simulink model "CiEngineController"  (R2017b)
settings: Solver=ode4  StartTime=0.0  StopTime=inf  FixedStep=.01  RelTol=1e-3  EnableMultiTasking=on
model workspace (MAT data in the model file):
  AFRStoich = 14.6
  CatLightOffTime = 0
  Cps = 2
  DesiredIdleSpeed = 750
  EGRAP_FFD = [31.29325855 19.51543729 10.79128083 10.46559436 21.98337597 33.12149522 39.82825957 47.90500302 59.68238122 67.88485049 66.83182002 60.43695561 ... (225 elements, 15x15)]
  EngStopStartEnable = 1
  EngStopTime = Simulink.Parameter
  EngStopTime.Value = 5
  EngStopTime.DataType = 'auto'
  EngStopTime.Dimensions = [1 1]
  InjSlp = 6.45161290323
  NCyl = 4
  Pstd = 101325
  Rair = 287.05
  Speed_bp = [1000 1285.71428571 1571.42857143 1857.14285714 2142.85714286 2428.57142857 2714.28571429 3000 3285.71428571 3571.42857143 3857.14285714 4142.85714286 4428.57142857 4714.28571429 5000]
  TQ_Simple = [0 10.3191931725 31.7529891947 50.7995054407 67.7372596761 83.6143476896 99.4031459341 115.400676238 131.426595678 147.347834106 163.740159238 181.145988166 ... (225 elements, 15x15)]
  TQ_Simple_FuelMass_bp = [0 3.5714 7.1429 10.7143 14.2857 17.8571 21.4286 25 28.5714 32.1429 35.7143 39.2857 42.8571 46.4286 50]
  TQ_Simple_Speed_bp = [1000 1410.7143 1821.4286 2232.1429 2642.8571 3053.5714 3464.2857 3875 4285.7143 4696.4286 5107.1429 5517.8571 5928.5714 6339.2857 6750]
  Torque_bp = [10 26.4285714286 42.8571428571 59.2857142857 75.7142857143 92.1428571429 108.571428571 125 141.428571429 157.857142857 174.285714286 190.714285714 207.142857143 223.571428571 240]
  Ts = Simulink.Parameter
  Ts.Value = 0.01
  Ts.DataType = 'auto'
  Ts.Dimensions = [1 1]
  Tstd = 293.15
  VGTPOS_FFD = [0.726426588 0.790379264 0.744536274 0.574005744 0.384541159 0.290234957 0.352244481 0.466398697 0.509945722 0.516364986 0.532540266 0.566278183 ... (225 elements, 15x15)]
  Vd = 0.0015
  VolEffEngSpdBpt = [1000 1285.71428571 1571.42857143 1857.14285714 2142.85714286 2428.57142857 2714.28571429 3000 3285.71428571 3571.42857143 3857.14285714 4142.85714286 4428.57142857 4714.28571429 5000]
  VolEffMapBpt = [95 100.344827586 105.689655172 111.034482759 116.379310345 121.724137931 127.068965517 132.413793103 137.75862069 143.103448276 148.448275862 153.793103448 159.137931034 164.482758621 169.827586207 175.172413793 180.517241379 185.862068966 191.206896552 196.551724138 201.896551724 207.24137931 212.586206897 217.931034483 223.275862069 228.620689655 233.965517241 239.310344828 244.655172414 250]
  VolEffTbl = [0.954646224834 0.927678310575 0.901063682417 0.875710037198 0.852450535311 0.831986822876 0.814844392337 0.80134438932 0.791593989181 0.785495277781 0.782770492696 0.782999798686 ... (450 elements, 30x15)]
  f_egr_stdflow = [0 0 0 0 0 0 0 0 0 0 0 0 ... (225 elements, 15x15)]
  f_egr_stdflow_egrap_bpt = [0 7.14285714286 14.2857142857 21.4285714286 28.5714285714 35.7142857143 42.8571428571 50 57.1428571429 64.2857142857 71.4285714286 78.5714285714 85.7142857143 92.8571428571 100]
  f_egr_stdflow_pr_bpt = [0.5 0.535714285714 0.571428571429 0.607142857143 0.642857142857 0.678571428571 0.714285714286 0.75 0.785714285714 0.821428571429 0.857142857143 0.892857142857 0.928571428571 0.964285714286 1]
  f_f_tot_n_bpt = [1000 1285.71428571 1571.42857143 1857.14285714 2142.85714286 2428.57142857 2714.28571429 3000 3285.71428571 3571.42857143 3857.14285714 4142.85714286 4428.57142857 4714.28571429 5000]
  f_f_tot_tq_bpt = [0 10 26.42857143 42.85714286 59.28571429 75.71428571 92.14285714 108.5714286 125 141.4285714 157.8571429 174.2857143 190.7142857 207.1428571 223.5714286 240]
  f_fcmd_tot = [7.10205580862 7.10205580862 10.8378455551 14.7842820505 18.9326887052 24.470710663 31.0466929023 35.2080453505 35.2080451224 35.2080448944 35.2080461396 35.2080459117 ... (240 elements, 16x15)]
  f_fric_temp_bpt = [275 277 279 281 283 285 287 289 291 293 295 297 299 301 303 305 307 309 311 313 315 317 319 321 323 325 327 329 331 333 335 337 339 341 343 345 347 349 351 353 355 357 359 361 363 365]
  f_fric_temp_mod = [3.986 2.616 2.132 1.946 1.839 1.747 1.672 1.608 1.551 1.499 1.462 1.415 1.363 1.314 1.275 1.248 1.223 1.195 1.173 1.15 1.134 1.113 1.097 1.082 1.065 1.051 1.039 1.025 1.01 1.001 0.9907 0.9802 0.9699 0.9595 0.9593 0.954 0.9415 0.9368 0.9285 0.923 0.9185 0.9093 0.9018 0.8989 0.8965 0.887]
  f_main_soi = [1.11993303174 2.12125793974 1.25580736048 -0.781894253933 -4.17418882707 -6.2159077095 -4.45741400372 -3.71779708796 -4.35326957016 -4.73674822365 -4.93672626877 -4.76868482083 ... (225 elements, 15x15)]
  f_main_soi_f_bpt = [3.57 6.855 10.14 13.425 16.71 19.995 23.28 26.565 29.85 33.135 36.42 39.705 42.99 46.275 49.56]
  f_main_soi_n_bpt = [1000 1285.71428571 1571.42857143 1857.14285714 2142.85714286 2428.57142857 2714.28571429 3000 3285.71428571 3571.42857143 3857.14285714 4142.85714286 4428.57142857 4714.28571429 5000]
  f_t_exh = [358.711368346 429.963145924 497.987869771 559.016510887 625.497016294 690.207854611 731.780908025 749.899407528 764.155922317 789.797182974 824.513264157 858.92580636 ... (240 elements, 16x15)]
  f_t_exh_f_bpt = [0 3.57 6.855 10.14 13.425 16.71 19.995 23.28 26.565 29.85 33.135 36.42 39.705 42.99 46.275 49.56]
  f_t_exh_n_bpt = [1000 1285.71428571 1571.42857143 1857.14285714 2142.85714286 2428.57142857 2714.28571429 3000 3285.71428571 3571.42857143 3857.14285714 4142.85714286 4428.57142857 4714.28571429 5000]
  f_tq_apc_bpt = [94.6146459029 109.976602506 125.338559109 140.700515712 156.062472315 171.424428919 186.786385522 202.148342125 217.510298728 232.872255331 248.234211934 263.596168537 278.958125141 294.320081744 309.682038347]
  f_tq_apc_mod = [0.999715885044 0.999538569407 0.999259905514 0.998809242093 0.998358578671 0.997880679846 0.997234389999 0.996588100153 0.995941810306 0.99547925674 0.995035391789 0.994591526839 ... (240 elements, 15x16)]
  f_tq_fric = [0  8.35  9.18  10  10.9  11.8  12.8  13.7  14.7  15.8  16.8  17.8  18.9  20  21.1  22.2; 0  8.35  9.18  10  10.9  11.8  12.8  13.7  14.7  15.8  16.8  17.8  18.9  20  21.1  22.2; 0  8.57  9.36  10.2  11.1  12  12.9  13.9  14.9  16  17  18.1  19.2  20.2  21.3  22.4; 0  8.79  9.56  10.4  11.2  12.2  13.1  14.1  15.2  16.2  17.3  18.4  19.5  20.6  21.6  22.7; 0  8.99  9.74  10.6  11.5  12.4  13.4  14.4  15.4  16.5  17.6  18.7  19.8  20.9  22  23.1; 0  9.19  9.94  10.8  11.7  12.7  13.7  14.7  15.8  16.8  17.9  19  20  21.1  22.3  23.4; 0  9.42  10.2  11  12  13.1  14.1  15.2  16.2  17.3  18.3  19.3  20.4  21.5  22.6  23.7; 0  9.7  10.4  11.3  12.4  13.5  14.6  15.7  16.8  17.9  18.9  19.9  21  22  23.1  24.1; 0  9.78  10.6  11.6  12.6  13.8  15  16.1  17.3  18.4  19.5  20.5  21.6  22.6  23.7  24.7; 0  9.84  10.8  11.7  12.8  13.9  15.1  16.3  17.5  18.6  19.7  20.8  21.9  23  24  25.1; 0  9.92  10.9  11.9  12.9  14.1  15.3  16.4  17.6  18.6  19.7  20.8  21.9  23  24.1  25.2; 0  10  11  12  13.1  14.3  15.5  16.7  17.8  18.8  19.9  20.9  22  23.1  24.2  25.4; 0  10.1  11.2  12.2  13.3  14.5  15.7  16.9  18.1  19.1  20.2  21.2  22.2  23.3  24.4  25.6; 0  10.3  11.3  12.3  13.4  14.6  15.7  16.9  18.1  19.2  20.3  21.3  22.4  23.4  24.6  25.7; 0  10.4  11.4  12.5  13.6  14.7  15.8  17  18.1  19.2  20.3  21.4  22.5  23.6  24.7  25.9; 0  10.5  11.6  12.6  13.7  14.8  15.9  17  18.2  19.3  20.4  21.5  22.6  23.7  24.8  26]
  f_tq_inr = [18.932941535 18.932941535 39.3255223176 57.8807366655 73.6414164249 90.1575991353 102.879416349 112.92944314 130.905512841 149.615511709 168.234721026 187.879026911 ... (256 elements, 16x16)]
  f_tq_inr_f_bpt = [0 3.57 6.855 10.14 13.425 16.71 19.995 23.28 26.565 29.85 33.135 36.42 39.705 42.99 46.275 49.56]
  f_tq_inr_n_bpt = [0 1000 1285.71428571 1571.42857143 1857.14285714 2142.85714286 2428.57142857 2714.28571429 3000 3285.71428571 3571.42857143 3857.14285714 4142.85714286 4428.57142857 4714.28571429 5000]
  f_tq_mainsoi_bpt = [-15 -13.7142857143 -12.4285714286 -11.1428571429 -9.85714285714 -8.57142857143 -7.28571428571 -6 -4.71428571429 -3.42857142857 -2.14285714286 -0.857142857143 0.428571428571 1.71428571429 3]
  f_tq_mainsoi_mod = [0.81078150005 0.827839263513 0.848673573925 0.874587588348 0.900164013454 0.923298328972 0.948048831471 0.970618714872 0.98831830141 0.997452724955 1 1 ... (240 elements, 15x16)]
  f_tq_map_bpt = [94.6146459029 109.976602506 125.338559109 140.700515712 156.062472315 171.424428919 186.786385522 202.148342125 217.510298728 232.872255331 248.234211934 263.596168537 278.958125141 294.320081744 309.682038347]
  f_tq_map_mod = [0.882177094009 0.934851504719 0.96634483908 0.97127123182 0.962954413121 0.952665164101 0.94513861625 0.942129377179 0.94335561462 0.947447812134 0.952949052459 0.958725491494 ... (240 elements, 15x16)]
  f_tq_mat_bpt = [35 42.8571428571 50.7142857143 58.5714285714 66.4285714286 74.2857142857 82.1428571429 90 97.8571428571 105.714285714 113.571428571 121.428571429 129.285714286 137.142857143 145]
  f_tq_mat_mod = [0.979193935333 0.989700620258 0.997707737278 1 0.992841543128 0.973230182048 0.94195882355 0.902873432246 0.86074346216 0.81947608235 0.779242235611 0.739783745312 ... (240 elements, 15x16)]
  f_tq_pump = [0  1  1  1.14  1.4  1.7  1.98  2.25  2.57  2.99  3.52  4.17  4.97  5.8  6.65  7.52; 0  1  1  1.14  1.4  1.7  1.98  2.25  2.57  2.99  3.52  4.17  4.97  5.8  6.65  7.52; 0  1  1  1.14  1.39  1.7  1.95  2.18  2.44  2.79  3.23  3.8  4.58  5.38  6.2  6.83; 0  1  1  1.11  1.32  1.7  2.05  2.37  2.7  3.03  3.4  3.83  4.45  5.19  6.02  6.74; 0  1  1  1.05  1.18  1.57  1.99  2.46  2.99  3.54  4.05  4.5  4.93  5.45  6.04  6.69; 0  1  1  1  1.03  1.31  1.64  2.04  2.6  3.3  4.01  4.67  5.2  5.73  6.3  7.01; 0  1  1  1.06  1.23  1.83  2.31  2.73  3.11  3.53  3.95  4.35  4.75  5.27  5.94  6.98; 0  1  1  1.21  1.7  3.02  4.17  5.18  5.95  6.49  6.85  6.98  6.84  6.8  6.92  7.67; 0  1  1  1  1.18  2.66  4.22  5.82  7.42  8.93  10.2  11.1  11.3  11.2  10.9  10.9; 0  1  1  1  1.06  1.51  2.69  4.26  6.02  7.9  9.71  11.4  12.4  13.2  13.6  13.9; 0  1  1  1  1  1  1.81  3.05  4.51  5.87  7.14  8.31  9.49  10.7  12.1  13.4; 0  1  1  1  1  1  1.43  2.28  3.79  4.97  5.92  6.63  7.49  8.67  10.2  12.2; 0  1  1  1  1  1  1.13  1.68  3.34  4.75  5.91  6.75  7.6  8.75  10.3  12.4; 0  1  1  1  1  1  1  1.38  2.91  4.49  5.87  6.9  7.77  9.05  10.8  13; 0  1  1  1  1  1  1  1.35  2.73  4.29  5.79  7.11  8.33  9.8  11.5  13.8; 0  1  1  1  1  1  1  1.36  2.78  4.33  5.88  7.38  8.91  10.6  12.4  14.6]
  f_turbo_pr = [1 1 1.00366494858 1.00841236661 1.01669032671 1.02766916175 1.04245504306 1.0631733336 1.08916626118 1.1150966519 1.13221323152 1.13265585874 ... (225 elements, 15x15)]
  f_turbo_pr_corrspd_bpt = [30 556.428571429 1082.85714286 1609.28571429 2135.71428571 2662.14285714 3188.57142857 3715 4241.42857143 4767.85714286 5294.28571429 5820.71428571 6347.14285714 6873.57142857 7400]
  f_turbo_pr_stdflow_bpt = [3 7.07142857143 11.1428571429 15.2142857143 19.2857142857 23.3571428571 27.4285714286 31.5 35.5714285714 39.6428571429 43.7142857143 47.7857142857 51.8571428571 55.9285714286 60]
  f_turbo_pr_vgtposcorr = [1.02855954111; 1.02335294047; 1.0182251931; 1.01353160145; 1.00975100162; 1.00744452152; 1.00702711526; 1.00854725935; 1.01183484525; 1.0163858771; 1.02148385659; 1.0270522279; 1.03306395358; 1.03926964489; 1.04548847114]
  f_turbo_pr_vgtposcorr_bpt = [0.1; 0.164285714286; 0.228571428571; 0.292857142857; 0.357142857143; 0.421428571429; 0.485714285714; 0.55; 0.614285714286; 0.678571428571; 0.742857142857; 0.807142857143; 0.871428571429; 0.935714285714; 1]
libraries: simulink x3, autolibengctrlr x1
(part 1 of 2)
settings Model: ModifiedByFormat=The MathWorks, Inc.  Creator=The MathWorks, Inc.  LastModifiedBy=The MathWorks, Inc.
settings DataIOCC: DSMLogging=off
settings CodeAppCC: StateflowObjectComments=on
settings GRTTargetCC: TargetLangStandard=C89/C90 (ANSI)
settings ConfigComp: CovMetricSettings=dsw  CovHtmlReporting=on  CovSaveCumulativeToWorkspaceVar=on  CovSaveSingleToWorkspaceVar=on  CovShowResultsExplorer=off  CovExternalEMLEnable=off

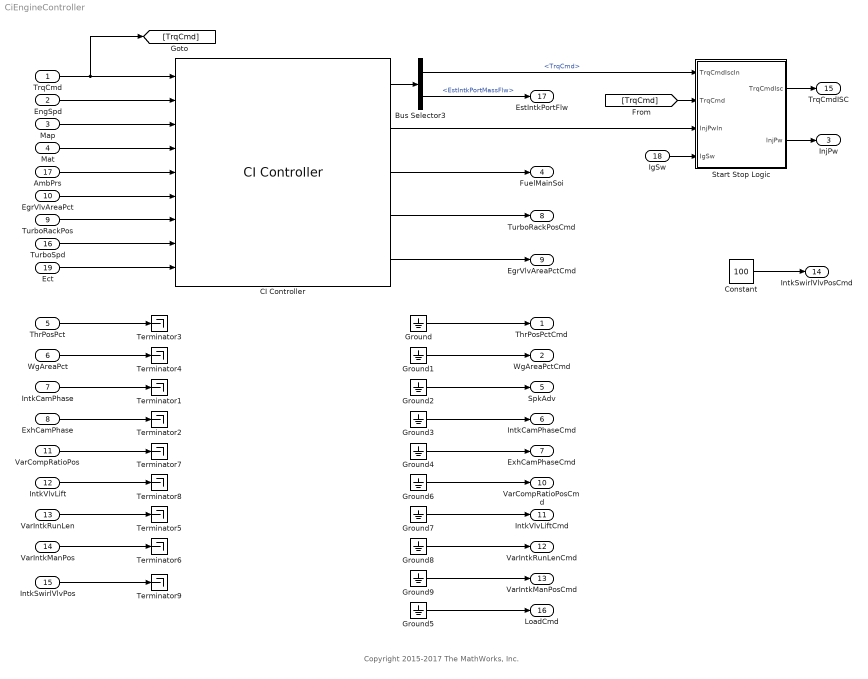
== system CiEngineController ==
  note: Copyright 2015-2017 The MathWorks, Inc.
  TrqCmd : Inport
  EngSpd : Inport  Port=2
  Map : Inport  Port=3
  Mat : Inport  Port=4
  ThrPosPct : Inport  Port=5  Unit=%
  WgAreaPct : Inport  Port=6  Unit=%
  IntkCamPhase : Inport  Port=7  Unit=deg
  ExhCamPhase : Inport  Port=8  Unit=deg
  TurboRackPos : Inport  Port=9
  EgrVlvAreaPct : Inport  Port=10
  VarCompRatioPos : Inport  Port=11
  IntkVlvLift : Inport  Port=12
  VarIntkRunLen : Inport  Port=13
  VarIntkManPos : Inport  Port=14
  IntkSwirlVlvPos : Inport  Port=15
  TurboSpd : Inport  Port=16
  AmbPrs : Inport  Port=17
  IgSw : Inport  Port=18
  Ect : Inport  Port=19  Unit=K
  Bus Selector3 : BusSelector  OutputSignals=TrqCmd,EstIntkPortMassFlw
  CI Controller : autolibengctrlr/CI Controller  TrqEstOptionPopup=Torque Structure  f_egrcmd=EGRAP_FFD  f_egr_tq_bpt=Torque_bp  f_egr_n_bpt=Speed_bp  f_rpcmd=VGTPOS_FFD  f_rp_tq_bpt=Torque_bp  f_rp_n_bpt=Speed_bp  Sinj=InjSlp  afr_stoich=AFRStoich  f_fcmd_tot=f_fcmd_tot  f_main_soi=f_main_soi  f_main_soi_f_bpt=f_main_soi_f_bpt  f_main_soi_n_bpt=f_main_soi_n_bpt  f_f_tot_tq_bpt=f_f_tot_tq_bpt  f_f_tot_n_bpt=f_f_tot_n_bpt  N_idle=DesiredIdleSpeed  Trq_idlecmd_enable=1  Trq_idlecmd_max=50  Kp_idle=0.1  Ki_idle=0.05  NCyl=NCyl  Cps=Cps  Vd=Vd  Rair=Rair  Pstd=Pstd  Tstd=Tstd  f_nv=VolEffTbl  f_nv_prs_bpt=VolEffMapBpt  f_nv_n_bpt=VolEffEngSpdBpt  f_egr_stdflow=f_egr_stdflow  f_egr_stdflow_pr_bpt=f_egr_stdflow_pr_bpt  f_egr_stdflow_egrap_bpt=f_egr_stdflow_egrap_bpt  f_turbo_pr=f_turbo_pr  f_turbo_pr_stdflow_bpt=f_turbo_pr_stdflow_bpt  f_turbo_pr_corrspd_bpt=f_turbo_pr_corrspd_bpt  f_turbo_pr_vgtposcorr=f_turbo_pr_vgtposcorr  f_turbo_pr_vgtposcorr_bpt=f_turbo_pr_vgtposcorr_bpt  f_tq_nf=TQ_Simple  f_tq_nf_f_bpt=TQ_Simple_FuelMass_bp  f_tq_nf_n_bpt=TQ_Simple_Speed_bp  f_tq_inr=f_tq_inr  f_tq_fric=f_tq_fric  f_fric_temp_mod=f_fric_temp_mod  f_fric_temp_bpt=f_fric_temp_bpt  f_tq_pump=f_tq_pump  f_tq_inr_f_bpt=f_tq_inr_f_bpt  f_tq_inr_n_bpt=f_tq_inr_n_bpt  f_tq_mainsoi_mod=f_tq_mainsoi_mod  f_tq_mainsoi_bpt=f_tq_mainsoi_bpt  f_tq_mat_mod=f_tq_mat_mod  f_tq_mat_bpt=f_tq_mat_bpt  f_tq_map_mod=f_tq_map_mod  f_tq_map_bpt=f_tq_map_bpt  f_tq_apc_mod=f_tq_apc_mod  f_tq_apc_bpt=f_tq_apc_bpt  f_t_exh=f_t_exh  f_t_exh_f_bpt=f_t_exh_f_bpt  f_t_exh_n_bpt=f_t_exh_n_bpt
      settings: SourceProductName=Powertrain Blockset  SourceProductBaseCode=PW
  Constant : Constant  Value=100
  Ground{,1..9} (10 alike) : Ground
  Start Stop Logic : Subsystem  TreatAsAtomicUnit=on
  Terminator{1..9} (9 alike) : Terminator
  ThrPosPctCmd : Outport  Unit=%
  WgAreaPctCmd : Outport  Port=2  Unit=%
  InjPw : Outport  Port=3  Unit=ms
  FuelMainSoi : Outport  Port=4
  SpkAdv : Outport  Port=5  Unit=deg
  IntkCamPhaseCmd : Outport  Port=6  Unit=deg
  ExhCamPhaseCmd : Outport  Port=7  Unit=deg
  TurboRackPosCmd : Outport  Port=8
  EgrVlvAreaPctCmd : Outport  Port=9
  VarCompRatioPosCmd : Outport  Port=10
  IntkVlvLiftCmd : Outport  Port=11
  VarIntkRunLenCmd : Outport  Port=12
  VarIntkManPosCmd : Outport  Port=13
  IntkSwirlVlvPosCmd : Outport  Port=14
  TrqCmdISC : Outport  Port=15  Unit=N*m
  LoadCmd : Outport  Port=16  Unit=1
  EstIntkPortFlw : Outport  Port=17  Unit=kg/s
  wires:
  AmbPrs/1 -> CI Controller/5
  Map/1 -> CI Controller/3
  Mat/1 -> CI Controller/4
  IntkCamPhase/1 -> Terminator1/1
  ExhCamPhase/1 -> Terminator2/1
  CI Controller/1 -> Bus Selector3/1
  EngSpd/1 -> CI Controller/2
  Ground/1 -> ThrPosPctCmd/1
  TrqCmd/1 -> [TrqCmd], CI Controller/1
  Bus Selector3/1 -> Start Stop Logic/1(TrqCmdIscIn)  "<TrqCmd>"
  CI Controller/4 -> TurboRackPosCmd/1
  CI Controller/5 -> EgrVlvAreaPctCmd/1
  Ground1/1 -> WgAreaPctCmd/1
  Ground2/1 -> SpkAdv/1
  Ground3/1 -> IntkCamPhaseCmd/1
  Ground4/1 -> ExhCamPhaseCmd/1
  Bus Selector3/2 -> EstIntkPortFlw/1  "<EstIntkPortMassFlw>"
  Ground5/1 -> LoadCmd/1
  CI Controller/3 -> FuelMainSoi/1
  EgrVlvAreaPct/1 -> CI Controller/6
  TurboRackPos/1 -> CI Controller/7
  TurboSpd/1 -> CI Controller/8
  CI Controller/2 -> Start Stop Logic/3(InjPwIn)
  Start Stop Logic/2(InjPw) -> InjPw/1
  [TrqCmd] -> Start Stop Logic/2(TrqCmd)
  Start Stop Logic/1(TrqCmdIsc) -> TrqCmdISC/1
  Ground6/1 -> VarCompRatioPosCmd/1
  Ground7/1 -> IntkVlvLiftCmd/1
  Ground8/1 -> VarIntkRunLenCmd/1
  Ground9/1 -> VarIntkManPosCmd/1
  Constant/1 -> IntkSwirlVlvPosCmd/1
  WgAreaPct/1 -> Terminator4/1
  ThrPosPct/1 -> Terminator3/1
  VarCompRatioPos/1 -> Terminator7/1
  IntkVlvLift/1 -> Terminator8/1
  VarIntkManPos/1 -> Terminator6/1
  VarIntkRunLen/1 -> Terminator5/1
  IntkSwirlVlvPos/1 -> Terminator9/1
  IgSw/1 -> Start Stop Logic/4(IgSw)
  Ect/1 -> CI Controller/9
